simulink library "FF_Library"  (R2024b)
settings: Solver=VariableStepAuto  StartTime=0.0  StopTime=10.0  RelTol=1e-3
undefined symbols (not defined in the file or in its folder): Slope1, Slope2
libraries: simulink x60
(part 3 of 4)

== system FF_Library/Memory/RSFlipFlop ==
  u1 : Inport
  u2 : Inport  Port=2
  0 : UnitDelay  SampleTime=-1  HasFrameUpgradeWarning=on
  Constant : Constant  Value=false
  Constant1 : Constant  Value=true
  NOT : Logic  Operator=NOT  AllPortsSameDT=off  OutDataTypeStr=boolean
  Switch : Switch  Criteria=u2 > Threshold  InputSameDT=off
  Switch1 : Switch  Criteria=u2 > Threshold  InputSameDT=off
  y1 : Outport
  y2 : Outport  Port=2
  wires:
  u2/1 -> Switch/2
  Constant/1 -> Switch/1
  Switch1/1 -> Switch/3
  u1/1 -> Switch1/2
  Constant1/1 -> Switch1/1
  0/1 -> Switch1/3
  Switch/1 -> NOT/1, 0/1, y1/1
  NOT/1 -> y2/1

== system FF_Library/Memory/SAMPLEANDHOLD_RE ==
  note: x_out
  note: y
  u : Inport
  E : Inport  Port=2
  R : Inport  Port=3
  IV : Inport  Port=4
  x_in : Inport  Port=5
  Functionality : Subsystem
  y : Terminator
  x_out : Outport
  wires:
  E/1 -> Functionality/2(E)
  Functionality/2(x_out) -> x_out/1
  u/1 -> Functionality/1(u)
  Functionality/1(y) -> y/1
  IV/1 -> Functionality/4(IV)
  R/1 -> Functionality/3(R)
  x_in/1 -> Functionality/5(x_in)

== system FF_Library/Memory/SRFlipFlop ==
  u1 : Inport
  u2 : Inport  Port=2
  0 : UnitDelay  SampleTime=-1  HasFrameUpgradeWarning=on
  Constant2 : Constant  Value=true
  Constant3 : Constant  Value=false
  NOT : Logic  Operator=NOT  AllPortsSameDT=off  OutDataTypeStr=boolean
  Switch : Switch  Criteria=u2 > Threshold  InputSameDT=off
  Switch1 : Switch  Criteria=u2 > Threshold  InputSameDT=off
  y1 : Outport
  y2 : Outport  Port=2
  wires:
  0/1 -> Switch1/3
  Constant2/1 -> Switch/1
  Constant3/1 -> Switch1/1
  Switch1/1 -> Switch/3
  Switch/1 -> NOT/1, 0/1, y1/1
  NOT/1 -> y2/1
  u1/1 -> Switch/2
  u2/1 -> Switch1/2

== system FF_Library/Memory/SlideMemory ==
  X : Inport
  En : Inport  Port=2
  num : Inport  Port=3
  Chart1 : Stateflow chart  TreatAsAtomicUnit=on
      settings: PortSchema="{\"entries\":[{\"content\":{\"sides\":[{\"content\":{\"connectorIds\":[\"In2\",\"In3\",\"In4\",\"In1\"]},\"type\":\"ConnectorPlacement.EquallySpacedRectSide\",\"uuid\":\"d8d21780-e643-4652-9c64-19f9f30af64f\"},{\"content\":{\"connectorIds\":[\"Out1\"],\"side\":\"RIGHT\"},\"type\":\"ConnectorPlacement.EquallySpacedRectSide\",\"uuid\":\"7d69bba5-0763-4300-b19b-47924509af48\"},{\"content\":{\"side\":\"TOP\"},\"type\":\"ConnectorPlacement.EquallySpacedRectSide\",\"uuid\":\"38e4f22a-6151-46b5-8f75-5e76d990d379\"}]},\"type\":\"ConnectorPlacement.EquallySpacedConnector\",\"uuid\":\"2f120d82-570f-4fc2-83ec-a719f4da1cbc\"}],\"packageUris\":[\"http://schema.mathworks.com/mf0/Connector/R2020b\"],\"version\":\"1.0\"}"
  Unit Delay : UnitDelay  SampleTime=-1  HasFrameUpgradeWarning=on
  A : Outport
  wires:
  X/1 -> Chart1/2(X)
  Unit Delay/1 -> Chart1/1(Y)
  Chart1/1(A) -> A/1, Unit Delay/1
  En/1 -> Chart1/3(En)
  num/1 -> Chart1/4(num)

== system FF_Library/Unit/degps2radps ==
  g : Inport
  Product : Product  OutDataTypeStr=single
  pi/180 : Constant  Value=0.01744  OutDataTypeStr=single
  mps2 : Outport
  wires:
  Product/1 -> mps2/1
  g/1 -> Product/1
  pi/180/1 -> Product/2

== system FF_Library/Unit/g2mps2 ==
  g : Inport
  Constant : Constant  Value=9.8  OutDataTypeStr=single
  Product : Product  OutDataTypeStr=single
  mps2 : Outport
  wires:
  Constant/1 -> Product/2
  g/1 -> Product/1
  Product/1 -> mps2/1

== system FF_Library/Unit/mm to m2 ==
  In2 : Inport
  CNST_ONET : Constant  Value=single(1000)  OutDataTypeStr=single
  Product : Product  Inputs=*/
  Out2 : Outport  VectorParamsAs1DForOutWhenUnconnected=off
  wires:
  CNST_ONET/1 -> Product/2
  In2/1 -> Product/1
  Product/1 -> Out2/1

== system FF_Library/Counter&Timer/COUNTDOWN_RE/Functionality ==
  E : Inport
  R : Inport  Port=2
  IV : Inport  Description=Initial value  Port=3
  x_in : Inport  Port=4
  Constant1 : Constant  Value=0  OutDataTypeStr=Inherit: Inherit via back propagation
  Constant2 : Constant  OutDataTypeStr=Inherit: Inherit via back propagation
  Constant3 : Constant  Value=0  OutDataTypeStr=Inherit: Inherit via back propagation
  Data Type Duplicate1 : DataTypeDuplicate  NumInputPorts=3
  Relational Operator : RelationalOperator  Operator=>  OutDataTypeStr=float('double')
  Relational Operator1 : RelationalOperator  Operator=>  OutDataTypeStr=float('double')
  Signal Conversion : SignalConversion  ConversionOutput=Contiguous copy  OverrideOpt=off
  Signal Conversion1 : SignalConversion  ConversionOutput=Contiguous copy  OverrideOpt=off
  Sum1 : Sum  Inputs=-+
  Switch1 : Switch  Criteria=u2 ~= 0  OutDataTypeStr=Inherit: Inherit via back propagation  SaturateOnIntegerOverflow=off
  Switch2 : Switch  Criteria=u2 ~= 0  OutDataTypeStr=Inherit: Inherit via back propagation  SaturateOnIntegerOverflow=off  InputSameDT=off
  Switch3 : Switch  Criteria=u2 ~= 0  OutDataTypeStr=Inherit: Inherit via back propagation  SaturateOnIntegerOverflow=off
  y : Outport
  x_out : Outport  Port=2
  x : Outport  Port=3
  wires:
  Signal Conversion/1 -> x_out/1
  Relational Operator1/1 -> y/1
  Constant3/1 -> Relational Operator1/2
  Switch3/1 -> Switch1/1
  Sum1/1 -> Switch3/1
  Constant2/1 -> Sum1/1
  Relational Operator/1 -> Switch3/2
  x_in/1 -> Switch1/3, Switch3/3, Relational Operator/1, Sum1/2, Data Type Duplicate1/3
  Constant1/1 -> Relational Operator/2
  E/1 -> Switch1/2
  Switch2/1 -> Signal Conversion/1, Relational Operator1/1, Data Type Duplicate1/1, Signal Conversion1/1
  Switch1/1 -> Switch2/3
  R/1 -> Switch2/2
  IV/1 -> Switch2/1, Data Type Duplicate1/2
  Signal Conversion1/1 -> x/1

== system FF_Library/Counter&Timer/COUNTUP_RE/Functionality ==
  E : Inport
  R : Inport  Port=2
  IV : Inport  Description=Initial value  Port=3
  x_in : Inport  Port=4
  Constant3 : Constant  OutDataTypeStr=Inherit: Inherit via back propagation
  Data Type Duplicate : DataTypeDuplicate  NumInputPorts=3
  Signal Conversion : SignalConversion  ConversionOutput=Contiguous copy  OverrideOpt=off
  Signal Conversion1 : SignalConversion  ConversionOutput=Contiguous copy  OverrideOpt=off
  Sum1 : Sum
  Switch1 : Switch  Criteria=u2 ~= 0  OutDataTypeStr=Inherit: Inherit via back propagation  SaturateOnIntegerOverflow=off
  Switch2 : Switch  Criteria=u2 ~= 0  OutDataTypeStr=Inherit: Inherit via back propagation  SaturateOnIntegerOverflow=off  InputSameDT=off
  y : Outport
  x_out : Outport  Port=2
  wires:
  Signal Conversion1/1 -> y/1
  Signal Conversion/1 -> x_out/1
  Constant3/1 -> Sum1/1
  x_in/1 -> Sum1/2, Switch1/3, Data Type Duplicate/3
  E/1 -> Switch1/2
  Switch2/1 -> Signal Conversion/1, Signal Conversion1/1, Data Type Duplicate/1
  Switch1/1 -> Switch2/3
  Sum1/1 -> Switch1/1
  IV/1 -> Switch2/1, Data Type Duplicate/2
  R/1 -> Switch2/2

== system FF_Library/Counter&Timer/TIMER_RE/Functionality ==
  E : Inport
  R : Inport  Port=2
  IV : Inport  Description=Initial value  Port=3
  dT : Inport  Port=4
  x_in : Inport  Port=5
  Constant : Constant  Value=0  OutDataTypeStr=Inherit: Inherit via back propagation
  Constant1 : Constant  Value=0  OutDataTypeStr=Inherit: Inherit via back propagation
  Constant2 : Constant  Value=0  OutDataTypeStr=Inherit: Inherit via back propagation
  Data Type Duplicate : DataTypeDuplicate  NumInputPorts=3
  Logical Operator : Logic  OutDataTypeStr=float('double')
  Relational Operator : RelationalOperator  Operator=<=  OutDataTypeStr=float('double')  InputSameDT=off
  Relational Operator1 : RelationalOperator  Operator=>  OutDataTypeStr=float('double')
  Relational Operator2 : RelationalOperator  Operator=>  OutDataTypeStr=float('double')  InputSameDT=off
  Signal Conversion : SignalConversion  ConversionOutput=Contiguous copy  OverrideOpt=off
  Sum1 : Sum  Inputs=+-
  Switch : Switch  Criteria=u2 ~= 0  OutDataTypeStr=Inherit: Inherit via back propagation  SaturateOnIntegerOverflow=off  InputSameDT=off
  Switch1 : Switch  Criteria=u2 ~= 0  OutDataTypeStr=Inherit: Inherit via back propagation  SaturateOnIntegerOverflow=off  InputSameDT=off
  Switch2 : Switch  Criteria=u2 ~= 0  OutDataTypeStr=Inherit: Inherit via back propagation  SaturateOnIntegerOverflow=off  InputSameDT=off
  y : Outport
  x_out : Outport  Port=2
  wires:
  Sum1/1 -> Switch2/1
  Switch2/1 -> Switch1/1
  Relational Operator2/1 -> Switch2/2
  Signal Conversion/1 -> x_out/1
  E/1 -> Switch1/2
  x_in/1 -> Sum1/1, Relational Operator2/1, Switch1/3, Data Type Duplicate/3, Relational Operator/1
  Constant/1 -> Relational Operator1/2
  Relational Operator1/1 -> y/1
  Switch/1 -> Signal Conversion/1, Relational Operator1/1, Data Type Duplicate/1
  Switch1/1 -> Switch/3
  Constant2/1 -> Switch2/3
  dT/1 -> Sum1/2, Relational Operator2/2
  IV/1 -> Switch/1, Data Type Duplicate/2
  Relational Operator/1 -> Logical Operator/2
  R/1 -> Logical Operator/1
  Logical Operator/1 -> Switch/2
  Constant1/1 -> Relational Operator/2

== system FF_Library/Counter&Timer/Timer/DIV ==
  In1 : Inport
  In2 : Inport  Port=2
  Constant2 : Constant  Value=abs(MinRange)  OutDataTypeStr=Inherit: Inherit via back propagation
  Constant3 : Constant  Value=-abs(MinRange)  OutDataTypeStr=Inherit: Inherit via back propagation
  Constant7 : Constant  Value=0  OutDataTypeStr=Inherit: Inherit via back propagation
  Divide1 : Product  Inputs=*/  SaturateOnIntegerOverflow=on
  Max2 : MinMax  Function=max  Inputs=2
  Min : MinMax  Inputs=2
  Relational Operator : RelationalOperator  OutDataTypeStr=boolean  RndMeth=Simplest  InputSameDT=off
  Switch : Switch  Criteria=u2 > Threshold  InputSameDT=off
  Out1 : Outport
  wires:
  Max2/1 -> Switch/1
  In2/1 -> Min/1, Max2/1, Relational Operator/1
  Constant7/1 -> Relational Operator/2
  Switch/1 -> Divide1/2
  Relational Operator/1 -> Switch/2
  Divide1/1 -> Out1/1
  In1/1 -> Divide1/1
  Constant2/1 -> Max2/2
  Min/1 -> Switch/3
  Constant3/1 -> Min/2

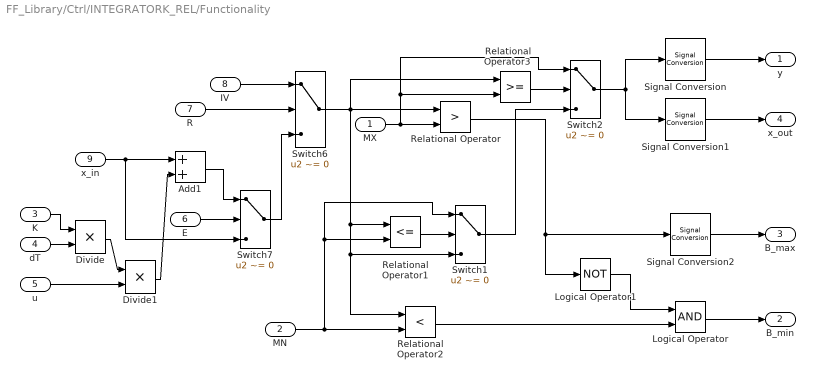
== system FF_Library/Ctrl/INTEGRATORK_REL/Functionality ==
  MX : Inport
  MN : Inport  Port=2
  K : Inport  Port=3
  dT : Inport  Port=4
  u : Inport  Port=5
  E : Inport  Port=6
  R : Inport  Port=7
  IV : Inport  Port=8
  x_in : Inport  Port=9
  Add1 : Sum
  Divide : Product  Inputs=**
  Divide1 : Product  Inputs=**
  Logical Operator : Logic  AllPortsSameDT=off  OutDataTypeStr=float('double')
  Logical Operator1 : Logic  Operator=NOT  AllPortsSameDT=off  OutDataTypeStr=float('double')
  Relational Operator : RelationalOperator  Operator=>  OutDataTypeStr=float('double')  InputSameDT=off
  Relational Operator1 : RelationalOperator  Operator=<=  OutDataTypeStr=float('double')  InputSameDT=off
  Relational Operator2 : RelationalOperator  Operator=<  OutDataTypeStr=float('double')  InputSameDT=off
  Relational Operator3 : RelationalOperator  OutDataTypeStr=float('double')  InputSameDT=off
  Signal Conversion : SignalConversion  ConversionOutput=Contiguous copy  OverrideOpt=off
  Signal Conversion1 : SignalConversion  ConversionOutput=Contiguous copy  OverrideOpt=off
  Signal Conversion2 : SignalConversion  ConversionOutput=Contiguous copy  OverrideOpt=off
  Switch1 : Switch  Criteria=u2 ~= 0  OutDataTypeStr=Inherit: Inherit via back propagation  SaturateOnIntegerOverflow=off  InputSameDT=off
  Switch2 : Switch  Criteria=u2 ~= 0  OutDataTypeStr=Inherit: Inherit via back propagation  SaturateOnIntegerOverflow=off  InputSameDT=off
  Switch6 : Switch  Criteria=u2 ~= 0  OutDataTypeStr=Inherit: Inherit via back propagation  SaturateOnIntegerOverflow=off
  Switch7 : Switch  Criteria=u2 ~= 0  OutDataTypeStr=Inherit: Inherit via back propagation  SaturateOnIntegerOverflow=off
  y : Outport
  B_min : Outport  Port=2
  B_max : Outport  Port=3
  x_out : Outport  Port=4
  wires:
  Switch1/1 -> Switch2/3
  Relational Operator3/1 -> Switch2/2
  Relational Operator1/1 -> Switch1/2
  Divide1/1 -> Add1/2
  u/1 -> Divide1/2
  Divide/1 -> Divide1/1
  Logical Operator/1 -> B_min/1
  Logical Operator1/1 -> Logical Operator/1
  Signal Conversion2/1 -> B_max/1
  R/1 -> Switch6/2
  IV/1 -> Switch6/1
  E/1 -> Switch7/2
  dT/1 -> Divide/2
  K/1 -> Divide/1
  x_in/1 -> Add1/1, Switch7/3
  Add1/1 -> Switch7/1
  Switch7/1 -> Switch6/3
  Switch6/1 -> Relational Operator/1, Switch1/3, Relational Operator2/1, Relational Operator1/1, Relational Operator3/1
  MX/1 -> Relational Operator/2, Relational Operator3/2, Switch2/1
  Relational Operator/1 -> Signal Conversion2/1, Logical Operator1/1
  MN/1 -> Relational Operator2/2, Switch1/1, Relational Operator1/2
  Relational Operator2/1 -> Logical Operator/2
  Switch2/1 -> Signal Conversion/1, Signal Conversion1/1
  Signal Conversion/1 -> y/1
  Signal Conversion1/1 -> x_out/1

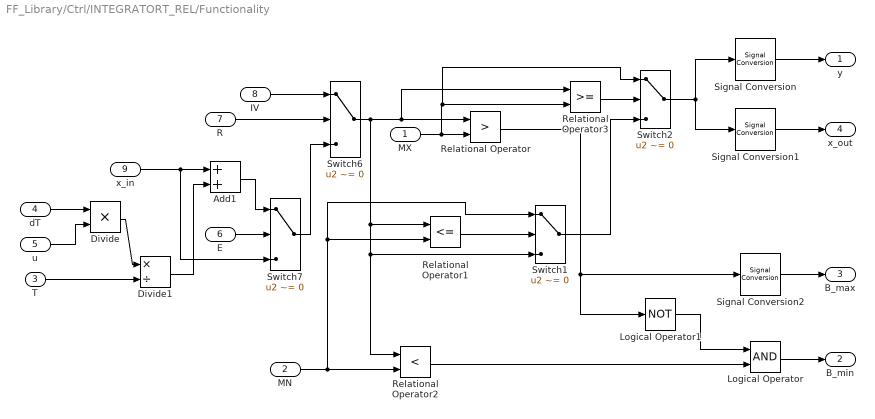
== system FF_Library/Ctrl/INTEGRATORT_REL/Functionality ==
  MX : Inport
  MN : Inport  Port=2
  T : Inport  Port=3
  dT : Inport  Port=4
  u : Inport  Port=5
  E : Inport  Port=6
  R : Inport  Port=7
  IV : Inport  Port=8
  x_in : Inport  Port=9
  Add1 : Sum
  Divide : Product  Inputs=**
  Divide1 : Product  Inputs=*/
  Logical Operator : Logic  AllPortsSameDT=off  OutDataTypeStr=float('double')
  Logical Operator1 : Logic  Operator=NOT  AllPortsSameDT=off  OutDataTypeStr=float('double')
  Relational Operator : RelationalOperator  Operator=>  OutDataTypeStr=float('double')  InputSameDT=off
  Relational Operator1 : RelationalOperator  Operator=<=  OutDataTypeStr=float('double')  InputSameDT=off
  Relational Operator2 : RelationalOperator  Operator=<  OutDataTypeStr=float('double')  InputSameDT=off
  Relational Operator3 : RelationalOperator  OutDataTypeStr=float('double')  InputSameDT=off
  Signal Conversion : SignalConversion  ConversionOutput=Contiguous copy  OverrideOpt=off
  Signal Conversion1 : SignalConversion  ConversionOutput=Contiguous copy  OverrideOpt=off
  Signal Conversion2 : SignalConversion  ConversionOutput=Contiguous copy  OverrideOpt=off
  Switch1 : Switch  Criteria=u2 ~= 0  OutDataTypeStr=Inherit: Inherit via back propagation  SaturateOnIntegerOverflow=off  InputSameDT=off
  Switch2 : Switch  Criteria=u2 ~= 0  OutDataTypeStr=Inherit: Inherit via back propagation  SaturateOnIntegerOverflow=off  InputSameDT=off
  Switch6 : Switch  Criteria=u2 ~= 0  OutDataTypeStr=Inherit: Inherit via back propagation  SaturateOnIntegerOverflow=off
  Switch7 : Switch  Criteria=u2 ~= 0  OutDataTypeStr=Inherit: Inherit via back propagation  SaturateOnIntegerOverflow=off
  y : Outport
  B_min : Outport  Port=2
  B_max : Outport  Port=3
  x_out : Outport  Port=4
  wires:
  Switch1/1 -> Switch2/3
  Relational Operator1/1 -> Switch1/2
  Relational Operator3/1 -> Switch2/2
  Divide1/1 -> Add1/2
  Divide/1 -> Divide1/1
  T/1 -> Divide1/2
  Signal Conversion2/1 -> B_max/1
  Logical Operator/1 -> B_min/1
  Logical Operator1/1 -> Logical Operator/1
  E/1 -> Switch7/2
  Switch2/1 -> Signal Conversion/1, Signal Conversion1/1
  R/1 -> Switch6/2
  IV/1 -> Switch6/1
  Switch7/1 -> Switch6/3
  x_in/1 -> Add1/1, Switch7/3
  Add1/1 -> Switch7/1
  Switch6/1 -> Relational Operator/1, Relational Operator3/1, Switch1/3, Relational Operator2/1, Relational Operator1/1
  MX/1 -> Relational Operator/2, Relational Operator3/2, Switch2/1
  Relational Operator/1 -> Signal Conversion2/1, Logical Operator1/1
  MN/1 -> Relational Operator2/2, Relational Operator1/2, Switch1/1
  Relational Operator2/1 -> Logical Operator/2
  dT/1 -> Divide/1
  u/1 -> Divide/2
  Signal Conversion/1 -> y/1
  Signal Conversion1/1 -> x_out/1

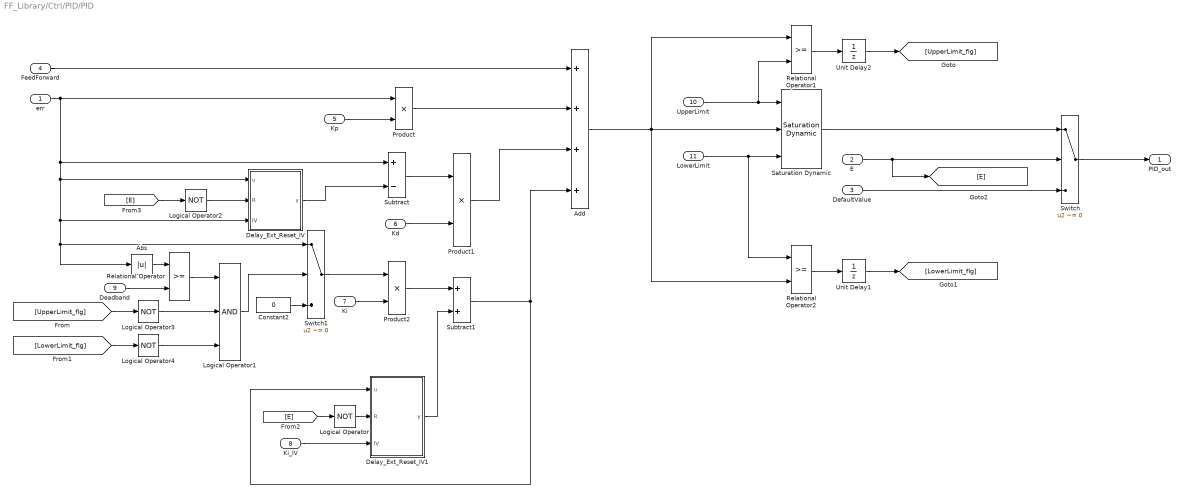
== system FF_Library/Ctrl/PID/PID ==
  err : Inport
  E : Inport  Port=2
  DefaultValue : Inport  Port=3
  FeedForward : Inport  Port=4
  Kp : Inport  Port=5
  Kd : Inport  Port=6
  Ki : Inport  Port=7
  Ki_IV : Inport  Port=8
  Deadband : Inport  Port=9
  UpperLimit : Inport  Port=10
  LowerLimit : Inport  Port=11
  Abs : Abs  RndMeth=Nearest
  Add : Sum  Inputs=++++  RndMeth=Nearest  SaturateOnIntegerOverflow=on
  Constant2 : Constant  Value=0  OutDataTypeStr=Inherit: Inherit via back propagation
      settings: AttributesFormatString=%<OutDataTypeStr>
  Delay_Ext_Reset_IV : Subsystem  mask(Delay_Ext_Reset_IV){}
      mask help:
      | 带Reset初始值功能的Delay模块：
      | 延迟输入u一个采样时间，初始值为IV；Reset后的输出y为IV。
      | u-输入值
      | IV-初始值
      | R-Reset标志
      | y-输出值
      mask Display: image('delay.GIF', [10,10,10,10,100,100]);
  Delay_Ext_Reset_IV1 : Subsystem  mask(Delay_Ext_Reset_IV){}
      mask help:
      | 带Reset初始值功能的Delay模块：
      | 延迟输入u一个采样时间，初始值为IV；Reset后的输出y为IV。
      | u-输入值
      | IV-初始值
      | R-Reset标志
      | y-输出值
      mask Display: image('delay.GIF', [10,10,10,10,100,100]);
  Logical Operator{,2..4} (4 alike) : Logic  Operator=NOT  AllPortsSameDT=off  OutDataTypeStr=boolean
  Logical Operator1 : Logic  Inputs=3  AllPortsSameDT=off  OutDataTypeStr=boolean
  Product : Product  RndMeth=Nearest  SaturateOnIntegerOverflow=on  OutDataTypeStr=Inherit: Same as first input
  Product1 : Product  RndMeth=Nearest  SaturateOnIntegerOverflow=on  OutDataTypeStr=Inherit: Same as first input
  Product2 : Product  RndMeth=Nearest  SaturateOnIntegerOverflow=on  OutDataTypeStr=Inherit: Same as first input
  Relational Operator : RelationalOperator  OutDataTypeStr=boolean  InputSameDT=off
  Relational Operator1 : RelationalOperator  OutDataTypeStr=boolean  InputSameDT=off
  Relational Operator2 : RelationalOperator  OutDataTypeStr=boolean  InputSameDT=off
  Saturation Dynamic : simulink/Discontinuities/Saturation Dynamic  OutMin=[]  OutMax=[]  OutDataTypeStr=Inherit: Same as second input  OutDataType=fixdt(1, 16)  OutScaling=2^-10  RndMeth=Nearest  DoSatur=off
  Subtract : Sum  Inputs=+-  RndMeth=Nearest  SaturateOnIntegerOverflow=on  OutDataTypeStr=Inherit: Same as first input
  Subtract1 : Sum  RndMeth=Nearest  SaturateOnIntegerOverflow=on  OutDataTypeStr=Inherit: Same as first input
  Switch : Switch  Criteria=u2 ~= 0  RndMeth=Nearest  InputSameDT=off
      settings: AttributesFormatString=%<Criteria>
  Switch1 : Switch  Criteria=u2 ~= 0  RndMeth=Nearest  InputSameDT=off
      settings: AttributesFormatString=%<Criteria>
  Unit Delay1 : UnitDelay  SampleTime=-1  HasFrameUpgradeWarning=on
      settings: AttributesFormatString=%<InitialCondition>
  Unit Delay2 : UnitDelay  SampleTime=-1  HasFrameUpgradeWarning=on
      settings: AttributesFormatString=%<InitialCondition>
  PID_out : Outport
  wires:
  Switch/1 -> PID_out/1
  E/1 -> [E], Switch/2
  DefaultValue/1 -> Switch/3
  Saturation Dynamic/1 -> Switch/1
  UpperLimit/1 -> Relational Operator1/2, Saturation Dynamic/1
  LowerLimit/1 -> Relational Operator2/1, Saturation Dynamic/3
  Add/1 -> Saturation Dynamic/2, Relational Operator2/2, Relational Operator1/1
  FeedForward/1 -> Add/1
  Product/1 -> Add/2
  err/1 -> Delay_Ext_Reset_IV/1(u), Delay_Ext_Reset_IV/3(IV), Switch1/1, Abs/1, Subtract/1, Product/1
  Kp/1 -> Product/2
  Delay_Ext_Reset_IV/1(y) -> Subtract/2
  Subtract/1 -> Product1/1
  Kd/1 -> Product1/2
  Product1/1 -> Add/3
  Ki/1 -> Product2/2
  Product2/1 -> Subtract1/1
  Delay_Ext_Reset_IV1/1(y) -> Subtract1/2
  Subtract1/1 -> Delay_Ext_Reset_IV1/1(u), Add/4
  Ki_IV/1 -> Delay_Ext_Reset_IV1/3(IV)
  Abs/1 -> Relational Operator/1
  Constant2/1 -> Switch1/3
  Switch1/1 -> Product2/1
  Deadband/1 -> Relational Operator/2
  Relational Operator1/1 -> Unit Delay2/1
  Relational Operator2/1 -> Unit Delay1/1
  [E] -> Logical Operator/1
  Logical Operator/1 -> Delay_Ext_Reset_IV1/2(R)
  Relational Operator/1 -> Logical Operator1/1
  Logical Operator1/1 -> Switch1/2
  [LowerLimit_flg] -> Logical Operator4/1
  [UpperLimit_flg] -> Logical Operator3/1
  Logical Operator3/1 -> Logical Operator1/2
  Logical Operator4/1 -> Logical Operator1/3
  [E] -> Logical Operator2/1
  Logical Operator2/1 -> Delay_Ext_Reset_IV/2(R)
  Unit Delay1/1 -> [LowerLimit_flg]
  Unit Delay2/1 -> [UpperLimit_flg]

== system FF_Library/Delay/TURNOFFDELAYSAMPLE/Functionality ==
  note: temp
  n : Inport
  u : Inport  Port=2
  R : Inport  Port=3
  x_in : Inport  Port=4
  Add1 : Sum  Inputs=+-
  Constant : Constant  Value=0  OutDataTypeStr=Inherit: Inherit via back propagation
  Constant1 : Constant  OutDataTypeStr=Inherit: Inherit via back propagation
  Data Type Duplicate : DataTypeDuplicate  NumInputPorts=3
  Logical Operator6 : Logic  Operator=OR  OutDataTypeStr=float('double')
  Relational Operator : RelationalOperator  Operator=>  OutDataTypeStr=float('double')  InputSameDT=off
  Signal Conversion : SignalConversion  ConversionOutput=Contiguous copy  OverrideOpt=off
  Switch1 : Switch  Criteria=u2 ~= 0  OutDataTypeStr=Inherit: Inherit via back propagation  SaturateOnIntegerOverflow=off
  Switch3 : Switch  Criteria=u2 ~= 0  OutDataTypeStr=Inherit: Inherit via back propagation  SaturateOnIntegerOverflow=off
  Switch4 : Switch  Criteria=u2 ~= 0  OutDataTypeStr=Inherit: Inherit via back propagation  SaturateOnIntegerOverflow=off
  y : Outport
  x_out : Outport  Port=2
  wires:
  R/1 -> Switch3/2
  n/1 -> Switch3/1, Switch1/1, Data Type Duplicate/3
  u/1 -> Switch1/2, Logical Operator6/1
  Constant/1 -> Relational Operator/2
  Relational Operator/1 -> Switch4/2, Logical Operator6/2
  x_in/1 -> Switch3/3, Data Type Duplicate/2, Switch4/3
  Constant1/1 -> Add1/2
  Switch3/1 -> Add1/1, Relational Operator/1
  Add1/1 -> Switch4/1
  Switch4/1 -> Switch1/3
  Logical Operator6/1 -> y/1
  Switch1/1 -> Signal Conversion/1, Data Type Duplicate/1
  Signal Conversion/1 -> x_out/1

== system FF_Library/Delay/TURNONDELAYSAMPLE/Functionality ==
  note: temp/x
  n : Inport
  u : Inport  Port=2
  R : Inport  Port=3
  x_in : Inport  Port=4
  Add1 : Sum  Inputs=+-
  Constant : Constant  OutDataTypeStr=Inherit: Inherit via back propagation
  Constant1 : Constant  Value=0  OutDataTypeStr=Inherit: Inherit via back propagation
  Constant3 : Constant  Value=0  OutDataTypeStr=Inherit: Inherit via back propagation
  Data Type Duplicate : DataTypeDuplicate  NumInputPorts=3
  Logical Operator : Logic  OutDataTypeStr=float('double')
  Relational Operator : RelationalOperator  Operator=>  OutDataTypeStr=float('double')  InputSameDT=off
  Relational Operator1 : RelationalOperator  Operator=<=  OutDataTypeStr=float('double')  InputSameDT=off
  Signal Conversion : SignalConversion  ConversionOutput=Contiguous copy  OverrideOpt=off
  Switch : Switch  Criteria=u2 ~= 0  OutDataTypeStr=Inherit: Inherit via back propagation  SaturateOnIntegerOverflow=off
  Switch1 : Switch  Criteria=u2 ~= 0  OutDataTypeStr=Inherit: Inherit via back propagation  SaturateOnIntegerOverflow=off  InputSameDT=off
  Switch2 : Switch  Criteria=u2 ~= 0  OutDataTypeStr=Inherit: Inherit via back propagation  SaturateOnIntegerOverflow=off
  y : Outport
  x_out : Outport  Port=2
  wires:
  Logical Operator/1 -> y/1
  Switch1/1 -> Signal Conversion/1, Data Type Duplicate/1
  n/1 -> Switch/1, Switch1/3, Data Type Duplicate/3
  u/1 -> Switch1/2, Logical Operator/1
  x_in/1 -> Switch/3, Data Type Duplicate/2
  R/1 -> Switch/2
  Switch/1 -> Add1/1, Relational Operator/1, Switch2/3, Relational Operator1/1
  Constant/1 -> Add1/2
  Add1/1 -> Switch2/1
  Relational Operator/1 -> Switch2/2
  Constant3/1 -> Relational Operator/2
  Switch2/1 -> Switch1/1
  Constant1/1 -> Relational Operator1/2
  Relational Operator1/1 -> Logical Operator/2
  Signal Conversion/1 -> x_out/1

== system FF_Library/Delay/TurnOffDeb/DIV1 ==
  In1 : Inport
  In2 : Inport  Port=2
  Constant2 : Constant  Value=abs(MinRange)  OutDataTypeStr=Inherit: Inherit via back propagation
  Constant3 : Constant  Value=-abs(MinRange)  OutDataTypeStr=Inherit: Inherit via back propagation
  Constant7 : Constant  Value=0  OutDataTypeStr=Inherit: Inherit via back propagation
  Divide1 : Product  Inputs=*/  SaturateOnIntegerOverflow=on
  Max2 : MinMax  Function=max  Inputs=2
  Min : MinMax  Inputs=2
  Relational Operator : RelationalOperator  OutDataTypeStr=boolean  RndMeth=Simplest  InputSameDT=off
  Switch : Switch  Criteria=u2 > Threshold  InputSameDT=off
  Out1 : Outport
  wires:
  Constant3/1 -> Min/2
  Min/1 -> Switch/3
  Constant2/1 -> Max2/2
  In1/1 -> Divide1/1
  Divide1/1 -> Out1/1
  Relational Operator/1 -> Switch/2
  Switch/1 -> Divide1/2
  Constant7/1 -> Relational Operator/2
  In2/1 -> Relational Operator/1, Max2/1, Min/1
  Max2/1 -> Switch/1

== system FF_Library/Delay/TurnOnDeb/DIV ==
  In1 : Inport
  In2 : Inport  Port=2
  Constant2 : Constant  Value=abs(MinRange)  OutDataTypeStr=Inherit: Inherit via back propagation
  Constant3 : Constant  Value=-abs(MinRange)  OutDataTypeStr=Inherit: Inherit via back propagation
  Constant7 : Constant  Value=0  OutDataTypeStr=Inherit: Inherit via back propagation
  Divide1 : Product  Inputs=*/  SaturateOnIntegerOverflow=on
  Max2 : MinMax  Function=max  Inputs=2
  Min : MinMax  Inputs=2
  Relational Operator : RelationalOperator  OutDataTypeStr=boolean  RndMeth=Simplest  InputSameDT=off
  Switch : Switch  Criteria=u2 > Threshold  InputSameDT=off
  Out1 : Outport
  wires:
  Max2/1 -> Switch/1
  In2/1 -> Min/1, Max2/1, Relational Operator/1
  Constant7/1 -> Relational Operator/2
  Switch/1 -> Divide1/2
  Relational Operator/1 -> Switch/2
  Divide1/1 -> Out1/1
  In1/1 -> Divide1/1
  Constant2/1 -> Max2/2
  Min/1 -> Switch/3
  Constant3/1 -> Min/2

== system FF_Library/Filter/DIGITALLOWPASS_RE/Functionality ==
  m : Inport
  u : Inport  Port=2
  E : Inport  Port=3
  R : Inport  Port=4
  IV : Inport  Port=5
  x_in : Inport  Port=6
  Add : Sum  Inputs=+-  InputSameDT=on  OutDataTypeStr=Inherit: Same as first input
  Add1 : Sum  InputSameDT=on  OutDataTypeStr=Inherit: Same as first input
  Product : Product  InputSameDT=on  OutDataTypeStr=Inherit: Same as first input
  Signal Conversion : SignalConversion  ConversionOutput=Contiguous copy  OverrideOpt=off
  Signal Conversion1 : SignalConversion  ConversionOutput=Contiguous copy  OverrideOpt=off
  Switch4 : Switch  Criteria=u2 ~= 0  OutDataTypeStr=Inherit: Inherit via back propagation  SaturateOnIntegerOverflow=off
  Switch6 : Switch  Criteria=u2 ~= 0  OutDataTypeStr=Inherit: Inherit via back propagation  SaturateOnIntegerOverflow=off
  y : Outport
  x_out : Outport  Port=2
  wires:
  R/1 -> Switch4/2
  IV/1 -> Switch4/1
  E/1 -> Switch6/2
  u/1 -> Add/1
  Add/1 -> Product/2
  m/1 -> Product/1
  Switch6/1 -> Switch4/3
  Switch4/1 -> Signal Conversion/1, Signal Conversion1/1
  Product/1 -> Add1/1
  x_in/1 -> Add1/2, Add/2, Switch6/3
  Add1/1 -> Switch6/1
  Signal Conversion/1 -> x_out/1
  Signal Conversion1/1 -> y/1

== system FF_Library/Filter/HIGHPASST_RE/Functionality ==
  T : Inport
  TD : Inport  Port=2
  dT : Inport  Port=3
  u : Inport  Port=4
  E : Inport  Port=5
  R : Inport  Port=6
  IV : Inport  Port=7
  x1_in : Inport  Port=8
  x2_in : Inport  Port=9
  Add : Sum
  Constant : Constant  OutDataTypeStr=Inherit: Inherit via back propagation
  DIV : Subsystem  mask(DIV){MinRange=1e-15}
      mask prompts: MinRange "smallest allowed value to divide by"
      mask help:
      | 除法模块：
      | 带有除0保护。
      mask Display:
      | port_label('input',1,'×');
      | port_label('input',2,'÷');
      | port_label('output',1,'');
  DIV1 : Subsystem  mask(DIV){MinRange=1e-15}
      mask prompts: MinRange "smallest allowed value to divide by"
      mask help:
      | 除法模块：
      | 带有除0保护。
      mask Display:
      | port_label('input',1,'×');
      | port_label('input',2,'÷');
      | port_label('output',1,'');
  Data Type Duplicate : DataTypeDuplicate
  Data Type Propagation : simulink/Signal Attributes/Data Type Propagation  PropDataType=sfix(16)  IfRefDouble=double  IfRefSingle=single  IsSigned=FALSE  NumBitsBase=NumBits1  NumBitsMult=0  NumBitsAdd=16  NumBitsAllowFinal=-1  PropScalingMode=Specify via dialog  PropScaling=2^-16  ValuesUsedBestPrec=[5 -7]  SlopeBase=min([Slope1 Slope2])  SlopeMult=1  SlopeAdd=0  BiasBase=Bias1  BiasMult=1  BiasAdd=0
  Divide : Product  Inputs=**
  Divide1 : Product  Inputs=**
  Signal Conversion : SignalConversion  ConversionOutput=Contiguous copy  OverrideOpt=off
  Signal Conversion1 : SignalConversion  ConversionOutput=Contiguous copy  OverrideOpt=off
  Signal Conversion2 : SignalConversion  ConversionOutput=Contiguous copy  OverrideOpt=off
  Sum1 : Sum  Inputs=+-
  Sum2 : Sum  Inputs=+-
  Switch4 : Switch  Criteria=u2 ~= 0  OutDataTypeStr=Inherit: Inherit via back propagation  SaturateOnIntegerOverflow=off
  Switch6 : Switch  Criteria=u2 ~= 0  OutDataTypeStr=Inherit: Inherit via back propagation  SaturateOnIntegerOverflow=off
  y : Outport
  x1_out : Outport  Port=2
  x2_out : Outport  Port=3
  wires:
  Signal Conversion2/1 -> x2_out/1
  Signal Conversion1/1 -> y/1
  Signal Conversion/1 -> x1_out/1
  R/1 -> Switch6/2
  IV/1 -> Data Type Duplicate/1, Switch6/1
  Switch6/1 -> Signal Conversion1/1, Signal Conversion/1
  Switch4/1 -> Switch6/3
  E/1 -> Switch4/2
  u/1 -> Sum2/1, Signal Conversion2/1
  dT/1 -> DIV/1(In1), Data Type Propagation/1
  Constant/1 -> Sum1/1
  DIV/1(Out1) -> Sum1/2, Data Type Propagation/3
  T/1 -> DIV/2(In2), DIV1/2(In2), Data Type Propagation/2
  TD/1 -> DIV1/1(In1)
  x2_in/1 -> Sum2/2
  DIV1/1(Out1) -> Divide/1
  Sum2/1 -> Divide/2
  Divide/1 -> Add/2
  Divide1/1 -> Add/1
  Sum1/1 -> Divide1/2
  Add/1 -> Switch4/1
  x1_in/1 -> Data Type Duplicate/2, Divide1/1, Switch4/3

== system FF_Library/Filter/LOWPASSK_RE/Functionality ==
  note: SDARevision: 8.4 $
      | library version information
  m : Inport
  u : Inport  Port=2
  E : Inport  Port=3
  R : Inport  Port=4
  IV : Inport  Port=5
  x_in : Inport  Port=6
  Add : Sum  InputSameDT=on  OutDataTypeStr=Inherit: Same as first input
  Add2 : Sum  Inputs=+-
  Data Type Duplicate : DataTypeDuplicate
  Product : Product  InputSameDT=on  OutDataTypeStr=Inherit: Same as first input
  Signal Conversion : SignalConversion  ConversionOutput=Contiguous copy  OverrideOpt=off
  Signal Conversion1 : SignalConversion  ConversionOutput=Contiguous copy  OverrideOpt=off
  Switch4 : Switch  Criteria=u2 ~= 0  OutDataTypeStr=Inherit: Inherit via back propagation  SaturateOnIntegerOverflow=off  InputSameDT=off
  Switch6 : Switch  Criteria=u2 ~= 0  SaturateOnIntegerOverflow=off
  y : Outport
  x_out : Outport  Port=2
  wires:
  Signal Conversion1/1 -> y/1
  Signal Conversion/1 -> x_out/1
  R/1 -> Switch4/2
  IV/1 -> Switch4/1
  E/1 -> Switch6/2
  x_in/1 -> Add2/2, Add/2, Switch6/3, Data Type Duplicate/2
  m/1 -> Product/1
  u/1 -> Add2/1
  Add2/1 -> Product/2
  Product/1 -> Add/1
  Switch6/1 -> Switch4/3
  Add/1 -> Switch6/1
  Switch4/1 -> Signal Conversion/1, Signal Conversion1/1, Data Type Duplicate/1

== system FF_Library/Filter/LOWPASSK_RE/check_mrange ==
  m : Inport
  Assertion : Assertion
  conjunction : Logic  OutDataTypeStr=float('double')
  max_relop : RelationalOperator  Operator=<  OutDataTypeStr=float('double')  InputSameDT=off
  max_val : Constant  OutDataTypeStr=int8
  min_relop : RelationalOperator  Operator=<=  OutDataTypeStr=float('double')  InputSameDT=off
  min_val : Constant  Value=0  OutDataTypeStr=int8
  out : Terminator
  wires:
  conjunction/1 -> Assertion/1, out/1
  max_relop/1 -> conjunction/2
  min_relop/1 -> conjunction/1
  max_val/1 -> max_relop/2
  min_val/1 -> min_relop/1
  m/1 -> max_relop/1, min_relop/2

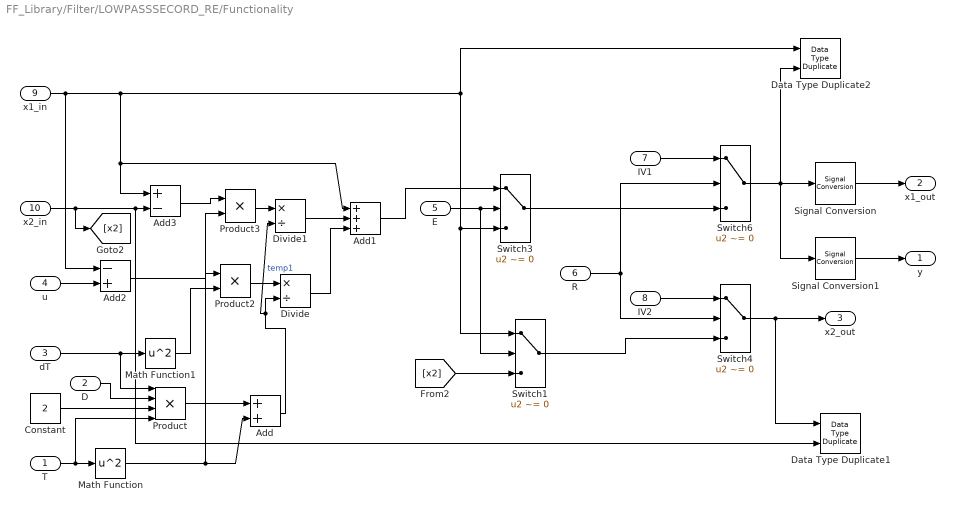
== system FF_Library/Filter/LOWPASSSECORD_RE/Functionality ==
  T : Inport
  D : Inport  Port=2
  dT : Inport  Port=3
  u : Inport  Port=4
  E : Inport  Port=5
  R : Inport  Port=6
  IV1 : Inport  Port=7
  IV2 : Inport  Port=8
  x1_in : Inport  Port=9
  x2_in : Inport  Port=10
  Add : Sum  InputSameDT=on  OutDataTypeStr=Inherit: Same as first input
  Add1 : Sum  Inputs=+++  InputSameDT=on  OutDataTypeStr=Inherit: Same as first input
  Add2 : Sum  Inputs=-+  InputSameDT=on  OutDataTypeStr=Inherit: Same as first input
  Add3 : Sum  Inputs=+-  InputSameDT=on  OutDataTypeStr=Inherit: Same as first input
  Constant : Constant  Value=2  OutDataTypeStr=Inherit: Inherit via back propagation
  Data Type Duplicate1 : DataTypeDuplicate
  Data Type Duplicate2 : DataTypeDuplicate
  Divide : Product  Inputs=*/  InputSameDT=on  OutDataTypeStr=Inherit: Same as first input
  Divide1 : Product  Inputs=*/  InputSameDT=on  OutDataTypeStr=Inherit: Same as first input
  Math Function : Math  Operator=square  SignedPower=on
  Math Function1 : Math  Operator=square  SignedPower=on
  Product : Product  Inputs=4  InputSameDT=on  OutDataTypeStr=Inherit: Same as first input
  Product2 : Product  InputSameDT=on  OutDataTypeStr=Inherit: Same as first input
  Product3 : Product  InputSameDT=on  OutDataTypeStr=Inherit: Same as first input
  Signal Conversion : SignalConversion  ConversionOutput=Contiguous copy  OverrideOpt=off
  Signal Conversion1 : SignalConversion  ConversionOutput=Contiguous copy  OverrideOpt=off
  Switch1 : Switch  Criteria=u2 ~= 0  SaturateOnIntegerOverflow=off
  Switch3 : Switch  Criteria=u2 ~= 0  SaturateOnIntegerOverflow=off
  Switch4 : Switch  Criteria=u2 ~= 0  OutDataTypeStr=Inherit: Inherit via back propagation  SaturateOnIntegerOverflow=off  InputSameDT=off
  Switch6 : Switch  Criteria=u2 ~= 0  OutDataTypeStr=Inherit: Inherit via back propagation  SaturateOnIntegerOverflow=off  InputSameDT=off
  y : Outport
  x1_out : Outport  Port=2
  x2_out : Outport  Port=3
  wires:
  Signal Conversion1/1 -> y/1
  Signal Conversion/1 -> x1_out/1
  R/1 -> Switch6/2, Switch4/2
  Switch6/1 -> Signal Conversion1/1, Data Type Duplicate2/2, Signal Conversion/1
  Switch4/1 -> x2_out/1, Data Type Duplicate1/1
  IV1/1 -> Switch6/1
  IV2/1 -> Switch4/1
  u/1 -> Add2/2
  T/1 -> Math Function/1, Product/4
  dT/1 -> Math Function1/1, Product/1
  Constant/1 -> Product/3
  D/1 -> Product/2
  Product/1 -> Add/1
  Math Function/1 -> Add/2, Product3/2
  x2_in/1 -> [x2], Add3/2, Data Type Duplicate1/2
  Add2/1 -> Product2/1
  Math Function1/1 -> Product2/2
  E/1 -> Switch3/2, Switch1/2
  Switch3/1 -> Switch6/3
  x1_in/1 -> Add3/1, Add1/1, Switch3/3, Switch1/1, Data Type Duplicate2/1, Add2/1
  Add3/1 -> Product3/1
  Divide1/1 -> Add1/2
  Divide/1 -> Add1/3
  Add1/1 -> Switch3/1
  [x2] -> Switch1/3
  Switch1/1 -> Switch4/3
  Product3/1 -> Divide1/1
  Product2/1 -> Divide/1
  Add/1 -> Divide/2, Divide1/2  "temp1"

== system FF_Library/Filter/LOWPASST_RE/Functionality ==
  m : Inport
  u : Inport  Port=2
  E : Inport  Port=3
  R : Inport  Port=4
  IV : Inport  Port=5
  x_in : Inport  Port=6
  Add : Sum  InputSameDT=on  OutDataTypeStr=Inherit: Same as first input
  Add2 : Sum  Inputs=+-  InputSameDT=on  OutDataTypeStr=Inherit: Same as first input
  Data Type Duplicate : DataTypeDuplicate
  Product : Product  OutDataTypeStr=Inherit: Inherit via back propagation  RndMeth=Zero
  Signal Conversion : SignalConversion  ConversionOutput=Contiguous copy  OverrideOpt=off
  Signal Conversion1 : SignalConversion  ConversionOutput=Contiguous copy  OverrideOpt=off
  Switch1 : Switch  Criteria=u2 ~= 0  OutDataTypeStr=Inherit: Inherit via back propagation  SaturateOnIntegerOverflow=off  InputSameDT=off
  Switch2 : Switch  Criteria=u2 ~= 0  SaturateOnIntegerOverflow=off
  y : Outport
  x_out : Outport  Port=2
  wires:
  Signal Conversion1/1 -> y/1
  Signal Conversion/1 -> x_out/1
  R/1 -> Switch1/2
  IV/1 -> Switch1/1
  Switch1/1 -> Signal Conversion/1, Signal Conversion1/1, Data Type Duplicate/1
  u/1 -> Add2/1
  x_in/1 -> Add/2, Switch2/3, Data Type Duplicate/2, Add2/2
  Add2/1 -> Product/2
  m/1 -> Product/1
  Add/1 -> Switch2/1
  E/1 -> Switch2/2
  Switch2/1 -> Switch1/3
  Product/1 -> Add/1

== system FF_Library/Filter/LOWPASST_RE/check_mrange ==
  m : Inport
  Assertion : Assertion
  conjunction : Logic  OutDataTypeStr=float('double')
  max_relop : RelationalOperator  Operator=<  OutDataTypeStr=float('double')  InputSameDT=off
  max_val : Constant  OutDataTypeStr=int8
  min_relop : RelationalOperator  Operator=<=  OutDataTypeStr=float('double')  InputSameDT=off
  min_val : Constant  Value=0  OutDataTypeStr=int8
  out : Terminator
  wires:
  conjunction/1 -> Assertion/1, out/1
  max_relop/1 -> conjunction/2
  min_relop/1 -> conjunction/1
  max_val/1 -> max_relop/2
  min_val/1 -> min_relop/1
  m/1 -> max_relop/1, min_relop/2

== system FF_Library/Filter/T-Filter/DIV1 ==
  In1 : Inport
  In2 : Inport  Port=2
  Constant2 : Constant  Value=abs(MinRange)  OutDataTypeStr=Inherit: Inherit via back propagation
  Constant3 : Constant  Value=-abs(MinRange)  OutDataTypeStr=Inherit: Inherit via back propagation
  Constant7 : Constant  Value=0  OutDataTypeStr=Inherit: Inherit via back propagation
  Divide1 : Product  Inputs=*/  SaturateOnIntegerOverflow=on
  Max2 : MinMax  Function=max  Inputs=2
  Min : MinMax  Inputs=2
  Relational Operator : RelationalOperator  OutDataTypeStr=boolean  RndMeth=Simplest  InputSameDT=off
  Switch : Switch  Criteria=u2 > Threshold  InputSameDT=off
  Out1 : Outport
  wires:
  Constant3/1 -> Min/2
  Min/1 -> Switch/3
  Constant2/1 -> Max2/2
  In1/1 -> Divide1/1
  Divide1/1 -> Out1/1
  Relational Operator/1 -> Switch/2
  Switch/1 -> Divide1/2
  Constant7/1 -> Relational Operator/2
  In2/1 -> Relational Operator/1, Max2/1, Min/1
  Max2/1 -> Switch/1

== system FF_Library/Limit/ACCUMULATOR_REL/Functionality ==
  MX : Inport
  MN : Inport  Port=2
  u : Inport  Port=3
  E : Inport  Port=4
  R : Inport  Port=5
  IV : Inport  Port=6
  x_in : Inport  Port=7
  Add1 : Sum
  Logical Operator : Logic  AllPortsSameDT=off  OutDataTypeStr=float('double')
  Logical Operator1 : Logic  Operator=NOT  AllPortsSameDT=off  OutDataTypeStr=float('double')
  Relational Operator : RelationalOperator  Operator=>  OutDataTypeStr=float('double')  InputSameDT=off
  Relational Operator1 : RelationalOperator  Operator=<=  OutDataTypeStr=float('double')  InputSameDT=off
  Relational Operator2 : RelationalOperator  Operator=<  OutDataTypeStr=float('double')  InputSameDT=off
  Relational Operator3 : RelationalOperator  OutDataTypeStr=float('double')  InputSameDT=off
  Signal Conversion : SignalConversion  ConversionOutput=Contiguous copy  OverrideOpt=off
  Signal Conversion1 : SignalConversion  ConversionOutput=Contiguous copy  OverrideOpt=off
  Signal Conversion2 : SignalConversion  ConversionOutput=Contiguous copy  OverrideOpt=off
  Switch1 : Switch  Criteria=u2 ~= 0  OutDataTypeStr=Inherit: Inherit via back propagation  SaturateOnIntegerOverflow=off
  Switch2 : Switch  Criteria=u2 ~= 0  OutDataTypeStr=Inherit: Inherit via back propagation  SaturateOnIntegerOverflow=off  InputSameDT=off
  Switch3 : Switch  Criteria=u2 ~= 0  OutDataTypeStr=Inherit: Inherit via back propagation  SaturateOnIntegerOverflow=off  InputSameDT=off
  Switch4 : Switch  Criteria=u2 ~= 0  OutDataTypeStr=Inherit: Inherit via back propagation  SaturateOnIntegerOverflow=off
  y : Outport
  B_min : Outport  Port=2
  B_max : Outport  Port=3
  x_out : Outport  Port=4
  wires:
  Switch2/1 -> Switch3/3
  Relational Operator3/1 -> Switch3/2
  Relational Operator1/1 -> Switch2/2
  Logical Operator/1 -> B_min/1
  Logical Operator1/1 -> Logical Operator/1
  Signal Conversion2/1 -> B_max/1
  Switch3/1 -> Signal Conversion/1, Signal Conversion1/1
  Relational Operator2/1 -> Logical Operator/2
  MN/1 -> Relational Operator2/2, Relational Operator1/2, Switch2/1
  Relational Operator/1 -> Logical Operator1/1, Signal Conversion2/1
  MX/1 -> Relational Operator/2, Relational Operator3/2, Switch3/1
  Switch1/1 -> Relational Operator/1, Relational Operator3/1, Switch2/3, Relational Operator2/1, Relational Operator1/1
  Switch4/1 -> Switch1/3
  Add1/1 -> Switch4/1
  x_in/1 -> Add1/1, Switch4/3
  u/1 -> Add1/2
  E/1 -> Switch4/2
  IV/1 -> Switch1/1
  R/1 -> Switch1/2
  Signal Conversion/1 -> x_out/1
  Signal Conversion1/1 -> y/1

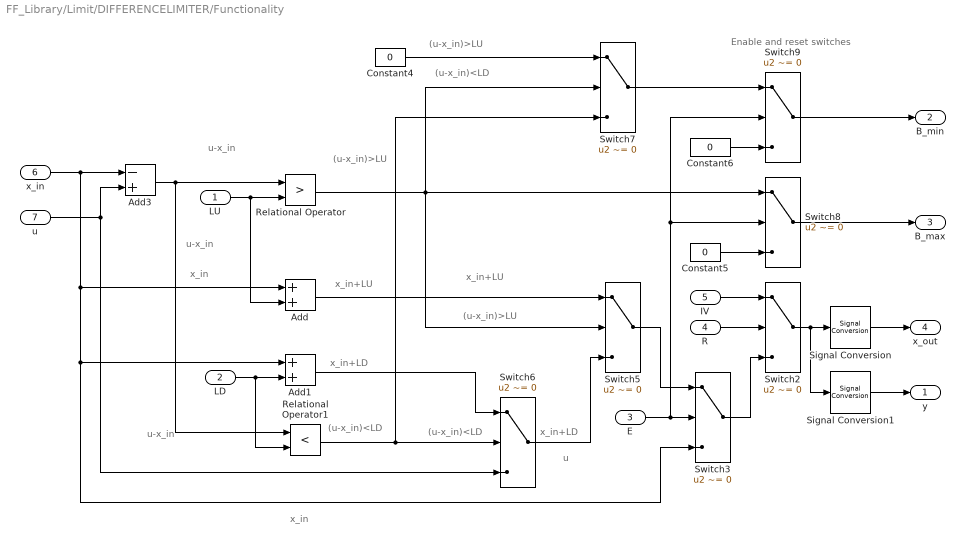
== system FF_Library/Limit/DIFFERENCELIMITER/Functionality ==
  note: x_in
  note: u-x_in
  note: x_in
  note: (u-x_in)<LD
  note: (u-x_in)>LU
  note: x_in+LU
  note: (u-x_in)<LD
  note: x_in+LD
  note: x_in+LU
  note: (u-x_in)>LU
  note: x_in+LD
  note: (u-x_in)<LD
  note: u
  note: (u-x_in)>LU
  note: u-x_in
  note: u-x_in
  note: Enable and reset switches
  LU : Inport
  LD : Inport  Port=2
  E : Inport  Port=3
  R : Inport  Port=4
  IV : Inport  Port=5
  x_in : Inport  Port=6
  u : Inport  Port=7
  Add : Sum
  Add1 : Sum
  Add3 : Sum  Inputs=-+
  Constant4 : Constant  Value=0  OutDataTypeStr=Inherit: Inherit via back propagation
  Constant5 : Constant  Value=0  OutDataTypeStr=Inherit: Inherit via back propagation
  Constant6 : Constant  Value=0  OutDataTypeStr=Inherit: Inherit via back propagation
  Relational Operator : RelationalOperator  Operator=>  OutDataTypeStr=float('double')  InputSameDT=off
  Relational Operator1 : RelationalOperator  Operator=<  OutDataTypeStr=float('double')  InputSameDT=off
  Signal Conversion : SignalConversion  ConversionOutput=Contiguous copy  OverrideOpt=off
  Signal Conversion1 : SignalConversion  ConversionOutput=Contiguous copy  OverrideOpt=off
  Switch{2..3,7..9} (5 alike) : Switch  Criteria=u2 ~= 0  OutDataTypeStr=Inherit: Inherit via back propagation  SaturateOnIntegerOverflow=off
  Switch5 : Switch  Criteria=u2 ~= 0  SaturateOnIntegerOverflow=off
  Switch6 : Switch  Criteria=u2 ~= 0  OutDataTypeStr=Inherit: Inherit via back propagation  SaturateOnIntegerOverflow=off  InputSameDT=off
  y : Outport
  B_min : Outport  Port=2
  B_max : Outport  Port=3
  x_out : Outport  Port=4
  wires:
  LD/1 -> Add1/2, Relational Operator1/2
  Switch9/1 -> B_min/1
  Constant6/1 -> Switch9/3
  Switch7/1 -> Switch9/1
  Constant5/1 -> Switch8/3
  Switch8/1 -> B_max/1
  Signal Conversion1/1 -> y/1
  Signal Conversion/1 -> x_out/1
  Constant4/1 -> Switch7/1
  Relational Operator/1 -> Switch5/2, Switch7/2, Switch8/1
  Relational Operator1/1 -> Switch6/2, Switch7/3
  x_in/1 -> Add3/1, Add/1, Add1/1, Switch3/3
  u/1 -> Add3/2, Switch6/3
  Add3/1 -> Relational Operator/1, Relational Operator1/1
  R/1 -> Switch2/2
  IV/1 -> Switch2/1
  Switch3/1 -> Switch2/3
  Switch2/1 -> Signal Conversion1/1, Signal Conversion/1
  E/1 -> Switch9/2, Switch8/2, Switch3/2
  Add/1 -> Switch5/1
  Add1/1 -> Switch6/1
  Switch5/1 -> Switch3/1
  Switch6/1 -> Switch5/3
  LU/1 -> Add/2, Relational Operator/2

== system FF_Library/Limit/DeadBan_RE/Functionality ==
  note: y
  note: u <= UMIN
  note: u - UMIN
  note: u - UMAX
  note: u >= UMAX
  UMAX : Inport
  UMIN : Inport  Port=2
  u : Inport  Port=3
  Add : Sum  Inputs=+-
  Add1 : Sum  Inputs=+-
  Relational Operator1 : RelationalOperator  Operator=<  OutDataTypeStr=float('double')  InputSameDT=off
  Relational Operator2 : RelationalOperator  Operator=<=  OutDataTypeStr=float('double')  InputSameDT=off
  Switch1 : Switch  Criteria=u2 ~= 0  Threshold=0.5  OutDataTypeStr=Inherit: Inherit via back propagation  SaturateOnIntegerOverflow=off
  Switch3 : Switch  Criteria=u2 ~= 0  Threshold=0.5  OutDataTypeStr=Inherit: Inherit via back propagation  SaturateOnIntegerOverflow=off
  ZERO1 : Constant  Value=0  OutDataTypeStr=Inherit: Inherit via back propagation
  y : Outport
  wires:
  Switch3/1 -> Switch1/3
  Add/1 -> Switch1/1
  Add1/1 -> Switch3/1
  ZERO1/1 -> Switch3/3
  Relational Operator2/1 -> Switch3/2
  Relational Operator1/1 -> Switch1/2
  u/1 -> Add1/1, Add/1, Relational Operator1/2, Relational Operator2/1
  Switch1/1 -> y/1
  UMAX/1 -> Add/2, Relational Operator1/1
  UMIN/1 -> Add1/2, Relational Operator2/2

== system FF_Library/Limit/DeadBand/Subsystem ==
  MX : Inport
  MN : Inport  Port=2
  u : Inport  Port=3
  AND : Logic  AllPortsSameDT=off  OutDataTypeStr=boolean
  Max1 : MinMax  Inputs=2  InputSameDT=on
  Max2 : MinMax  Function=max  Inputs=2  InputSameDT=on
  Relational Operator1 : RelationalOperator  Operator=<=  OutDataTypeStr=boolean  RndMeth=Simplest
  Relational Operator2 : RelationalOperator  Operator=<=  OutDataTypeStr=boolean  RndMeth=Simplest
  y : Outport
  wires:
  u/1 -> Relational Operator1/1, Relational Operator2/2
  Relational Operator2/1 -> AND/2
  Relational Operator1/1 -> AND/1
  MN/1 -> Max2/2, Max1/1
  Max2/1 -> Relational Operator1/2
  MX/1 -> Max2/1, Max1/2
  Max1/1 -> Relational Operator2/1
  AND/1 -> y/1

== system FF_Library/Limit/GRADIENTLIMITER/Functionality ==
  LU : Inport
  LD : Inport  Port=2
  dT : Inport  Port=3
  u : Inport  Port=4
  E : Inport  Port=5
  R : Inport  Port=6
  IV : Inport  Port=7
  x_in : Inport  Port=8
  Add2 : Sum  Inputs=-+
  Constant5 : Constant  Value=0  OutDataTypeStr=Inherit: Inherit via back propagation
  Constant6 : Constant  Value=0  OutDataTypeStr=Inherit: Inherit via back propagation
  Divide : Product  Inputs=**
  Divide1 : Product  Inputs=**
  Signal Conversion : SignalConversion  ConversionOutput=Contiguous copy  OverrideOpt=off
  Signal Conversion1 : SignalConversion  ConversionOutput=Contiguous copy  OverrideOpt=off
  Subfunctionality : Subsystem  mask(Subfunctionality_GRADIENTLIMITER_SIMULINK){}
  Switch8 : Switch  Criteria=u2 ~= 0  OutDataTypeStr=Inherit: Inherit via back propagation  SaturateOnIntegerOverflow=off
  Switch9 : Switch  Criteria=u2 ~= 0  OutDataTypeStr=Inherit: Inherit via back propagation  SaturateOnIntegerOverflow=off
  y : Outport
  B_min : Outport  Port=2
  B_max : Outport  Port=3
  x_out : Outport  Port=4
  wires:
  Divide1/1 -> Subfunctionality/2(LDdT)
  Divide/1 -> Subfunctionality/1(LUdT)
  LU/1 -> Divide/1
  LD/1 -> Divide1/1
  Subfunctionality/2(Bmin) -> Switch9/1
  Subfunctionality/1(Bmax) -> Switch8/1
  R/1 -> Subfunctionality/7(R)
  IV/1 -> Subfunctionality/6(IV)
  Add2/1 -> Subfunctionality/4(diff_ux)
  Subfunctionality/3(x_out) -> Signal Conversion1/1, Signal Conversion/1
  E/1 -> Switch9/2, Switch8/2, Subfunctionality/8(E)
  dT/1 -> Divide/2, Divide1/2
  Switch9/1 -> B_min/1
  Constant6/1 -> Switch9/3
  Constant5/1 -> Switch8/3
  Switch8/1 -> B_max/1
  Signal Conversion1/1 -> y/1
  Signal Conversion/1 -> x_out/1
  x_in/1 -> Add2/1, Subfunctionality/3(x_in)
  u/1 -> Add2/2, Subfunctionality/5(u)

== system FF_Library/Memory/BooleanHold/Count ==
  u : Inport
  Edge : Inport  Port=2
  Add : Sum  SaturateOnIntegerOverflow=on
  Logical Operator1 : Logic  OutDataTypeStr=boolean
  Logical Operator2 : Logic  Operator=NAND  OutDataTypeStr=boolean
  Logical Operator3 : Logic  Operator=NOT  AllPortsSameDT=off  OutDataTypeStr=boolean
  ONE : Constant  InitFcn=ONE=1;  OutDataTypeStr=uint16
  Relational Operator2 : RelationalOperator  Operator=~=  OutDataTypeStr=boolean  RndMeth=Simplest
  Relational Operator3 : RelationalOperator  OutDataTypeStr=boolean  RndMeth=Simplest
  Relational Operator4 : RelationalOperator  OutDataTypeStr=boolean  RndMeth=Simplest
  Switch : Switch  Criteria=u2 > Threshold  InputSameDT=off
  Switch1 : Switch  Criteria=u2 > Threshold  InputSameDT=off
  Unit_Delay : UnitDelay  SampleTime=-1  HasFrameUpgradeWarning=on
      settings: AttributesFormatString=init=%<X0>
  Unit_Delay2 : UnitDelay  SampleTime=-1  HasFrameUpgradeWarning=on
      settings: AttributesFormatString=init=%<X0>
  ZERO : Constant  InitFcn=ZERO=0;  Value=0  OutDataTypeStr=uint16
  ZERO1 : Constant  InitFcn=ZERO=0;  Value=True_Thd  OutDataTypeStr=uint16
  ZERO2 : Constant  InitFcn=ZERO=0;  Value=False_Thd  OutDataTypeStr=uint16
  TRUE_debounce : Outport
  FALSE_debounce : Outport  Port=2
  wires:
  ONE/1 -> Add/1
  ZERO/1 -> Switch/1
  u/1 -> Logical Operator1/1, Relational Operator2/1, Logical Operator3/1, Unit_Delay/1
  Switch1/1 -> Switch/3
  Unit_Delay2/1 -> Add/2, Switch1/3
  Unit_Delay/1 -> Relational Operator2/2
  Edge/1 -> Switch1/2
  Relational Operator2/1 -> Switch/2
  Switch/1 -> Unit_Delay2/1, Relational Operator4/1, Relational Operator3/1
  Add/1 -> Switch1/1
  ZERO1/1 -> Relational Operator3/2
  ZERO2/1 -> Relational Operator4/2
  Relational Operator3/1 -> Logical Operator1/2
  Relational Operator4/1 -> Logical Operator2/1
  Logical Operator3/1 -> Logical Operator2/2
  Logical Operator1/1 -> TRUE_debounce/1
  Logical Operator2/1 -> FALSE_debounce/1

== system FF_Library/Memory/DELTAONESTEP/Functionality ==
  u : Inport
  R : Inport  Port=2
  IV : Inport  Port=3
  x_in : Inport  Port=4
      settings: LatchInputForFeedbackSignals=on
  Trigger : TriggerPort  TriggerType=function-call  VariantControl=Variant  PortDimensions=1
  Add : Sum  Inputs=-+
  Data Type Duplicate : DataTypeDuplicate  NumInputPorts=3
  Signal Conversion : SignalConversion  ConversionOutput=Contiguous copy  OverrideOpt=off
  Switch : Switch  Criteria=u2 ~= 0  OutDataTypeStr=Inherit: Inherit via back propagation  SaturateOnIntegerOverflow=off  InputSameDT=off
  y : Outport
  x_out : Outport  Port=2
  wires:
  Add/1 -> y/1
  Switch/1 -> Add/1
  u/1 -> Add/2, Data Type Duplicate/1, Signal Conversion/1
  x_in/1 -> Data Type Duplicate/2, Switch/3
  IV/1 -> Data Type Duplicate/3, Switch/1
  R/1 -> Switch/2
  Signal Conversion/1 -> x_out/1

== system FF_Library/Memory/DIFFERENCEQUOTIENT/Functionality ==
  dT : Inport
  u : Inport  Port=2
  R : Inport  Port=3
  IV : Inport  Port=4
  x_in : Inport  Port=5
      settings: LatchInputForFeedbackSignals=on
  Trigger : TriggerPort  TriggerType=function-call  VariantControl=Variant  PortDimensions=1
  Add1 : Sum  Inputs=-+
  Data Type Conversion1 : DataTypeConversion  RndMeth=Floor
  Divide : Product  Inputs=*/
  Signal Conversion : SignalConversion  ConversionOutput=Contiguous copy  OverrideOpt=off
  Switch : Switch  Criteria=u2 ~= 0  OutDataTypeStr=Inherit: Inherit via back propagation  SaturateOnIntegerOverflow=off  InputSameDT=off
  y : Outport
  x_out : Outport  Port=2
  wires:
  Signal Conversion/1 -> Data Type Conversion1/1
  Add1/1 -> Divide/1
  Switch/1 -> Add1/1
  Divide/1 -> y/1
  dT/1 -> Divide/2
  u/1 -> Add1/2, Signal Conversion/1
  x_in/1 -> Switch/3
  IV/1 -> Switch/1
  R/1 -> Switch/2
  Data Type Conversion1/1 -> x_out/1
